simulink model "Inner4"  (Simulink 8.7)
settings: Solver=FixedStepDiscrete  StartTime=0.0  StopTime=20  RelTol=1e-3
settings Model: Creator=scaife  LastModifiedBy=bourbouh  ExtModeAutoUpdateStatusClock=off
settings DataIOCC: SignalLoggingSaveFormat=ModelDataLogs  SignalLoggingName=sigsOut
settings DebuggingCC: SaveWithParameterizedLinksMsg=none  SignalResolutionControl=TryResolveAllWithWarning  MultiTaskDSMMsg=warning  MultiTaskCondExecSysMsg=none
settings HardwareCC: TargetUnknown=on
settings SFSimCC: SimParseCustomCode=off
settings GRTTargetCC: CombineOutputUpdateFcns=off  GRTInterface=on

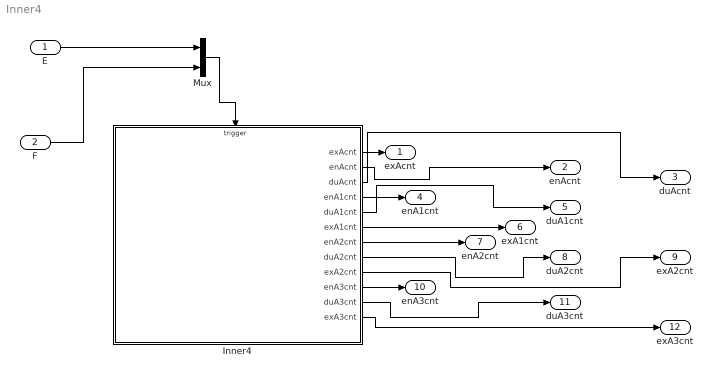
== system Inner4 ==
  E : Inport
  F : Inport  Port=2
  Inner4 : Stateflow chart  TreatAsAtomicUnit=on
  Mux : Mux  Inputs=2
  exAcnt : Outport
  enAcnt : Outport  Port=2
  duAcnt : Outport  Port=3
  enA1cnt : Outport  Port=4
  duA1cnt : Outport  Port=5
  exA1cnt : Outport  Port=6
  enA2cnt : Outport  Port=7
  duA2cnt : Outport  Port=8
  exA2cnt : Outport  Port=9
  enA3cnt : Outport  Port=10
  duA3cnt : Outport  Port=11
  exA3cnt : Outport  Port=12
  wires:
  Mux/1 -> Inner4/Trigger
  E/1 -> Mux/1
  F/1 -> Mux/2
  Inner4/1(exAcnt) -> exAcnt/1
  Inner4/2(enAcnt) -> enAcnt/1
  Inner4/3(duAcnt) -> duAcnt/1
  Inner4/4(enA1cnt) -> enA1cnt/1
  Inner4/5(duA1cnt) -> duA1cnt/1
  Inner4/6(exA1cnt) -> exA1cnt/1
  Inner4/7(enA2cnt) -> enA2cnt/1
  Inner4/8(duA2cnt) -> duA2cnt/1
  Inner4/9(exA2cnt) -> exA2cnt/1
  Inner4/12(exA3cnt) -> exA3cnt/1
  Inner4/10(enA3cnt) -> enA3cnt/1
  Inner4/11(duA3cnt) -> duA3cnt/1

== stateflow chart Inner4 ==
  state A/
    en: enAcnt++;
    du: duAcnt++;
    ex: exAcnt++;
    state A1/
      en: enA1cnt++;
      du: duA1cnt++;
      ex: exA1cnt++;
    state A2/
      en: enA2cnt++;
      du: duA2cnt++;
      ex: exA2cnt++;
    state A3/
      en: enA3cnt++;
      du: duA3cnt++;
      ex: exA3cnt++;
    (junction 7) -> A
    A1 -> (junction 7) [order 1] : E
    A3 -> (junction 7) [order 1] : E
    A2 -> (junction 7) [order 1] : E
    (default) -> A1
    A1 -> A2 [order 2] : F
    A2 -> A3 [order 2] : F
    A3 -> A1 [order 2] : F
  (default) -> A
  data: exAcnt output int32; enAcnt output int32; duAcnt output int32; enA1cnt output int32; duA1cnt output int32; exA1cnt output int32; enA2cnt output int32; duA2cnt output int32; exA2cnt output int32; enA3cnt output int32; duA3cnt output int32; exA3cnt output int32
  events: E input EITHER_EDGE_EVENT; F input EITHER_EDGE_EVENT
